simulink subsystem "VehicleAngularVelocity"  (R2024a)
settings: Solver=VariableStepAuto  StartTime=0.0  StopTime=10.0  RelTol=1e-3
libraries: uavmavlinklib x1
settings Model: Creator=gurt1  LastModifiedBy=gurt1

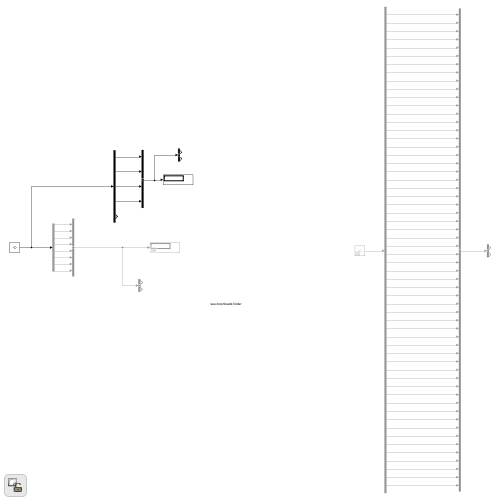
[thumbnail: Simulink's stored preview of the top-level diagram]
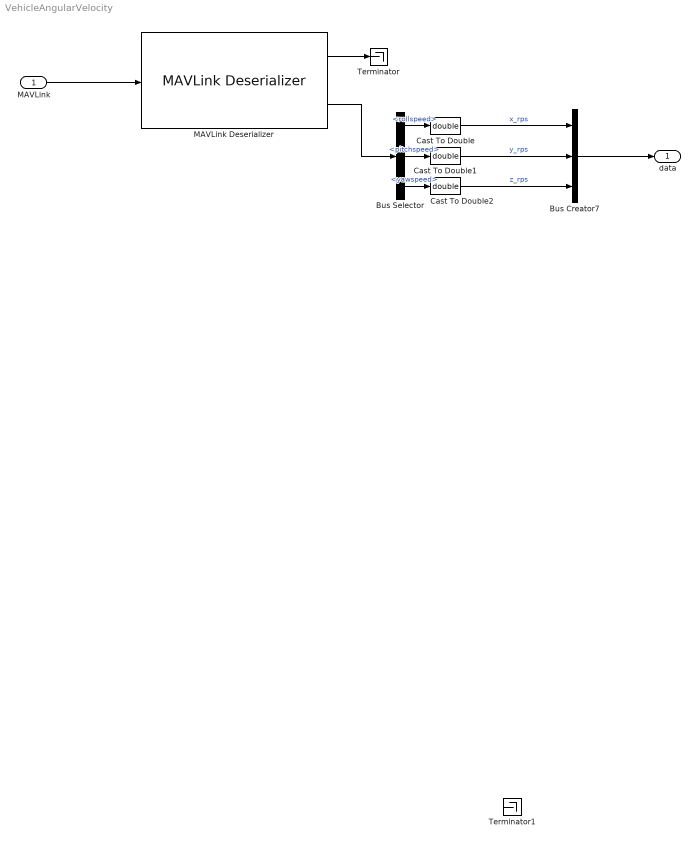
== system VehicleAngularVelocity ==
  MAVLink : Inport
  Bus Creator7 : BusCreator  Inputs=3
  Bus Selector : BusSelector  OutputSignals=Payload.rollspeed,Payload.pitchspeed,Payload.yawspeed
  Cast To Double : DataTypeConversion  OutDataTypeStr=double  SaturateOnIntegerOverflow=off  RndMeth=Floor
  Cast To Double1 : DataTypeConversion  OutDataTypeStr=double  SaturateOnIntegerOverflow=off  RndMeth=Floor
  Cast To Double2 : DataTypeConversion  OutDataTypeStr=double  SaturateOnIntegerOverflow=off  RndMeth=Floor
  MAVLink Deserializer : uavmavlinklib/MAVLink Deserializer  dialectSource=Select from standard MAVLink dialects  dialect=common.xml  dialectCustom=common.xml  version=2  messageType=ATTITUDE  inputDataLength=off  SystemIDFilter=off  systemID=1  ComponentIDFilter=off  componentID=1  queueMsg=off  queueMsgSize=50  dropNum=off
  Terminator : Terminator
  Terminator1 : Terminator
  data : Outport
  wires:
  ? -> ?
  Bus Creator7/1 -> data/1
  MAVLink/1 -> MAVLink Deserializer/1
  MAVLink Deserializer/1 -> Terminator/1
  MAVLink Deserializer/2 -> Bus Selector/1
  Bus Selector/1 -> Cast To Double/1  "<rollspeed>"
  Bus Selector/2 -> Cast To Double1/1  "<pitchspeed>"
  Bus Selector/3 -> Cast To Double2/1  "<yawspeed>"
  Cast To Double/1 -> Bus Creator7/1  "x_rps"
  Cast To Double1/1 -> Bus Creator7/2  "y_rps"
  Cast To Double2/1 -> Bus Creator7/3  "z_rps"
